simulink model "roll_lqt"  (R2022a)
settings: Solver=ode4  StartTime=0.0  StopTime=26  FixedStep=0.05  RelTol=1e-3
values from neighbouring files (symbols this model uses):
  B = [0 ... (first row only)    [LQR_solver.m]    (also in LQT_solver.m)
  K = ks(1:n, :)    [LQR_solver.m]    (also in LQT_solver.m)
  R_inv = 1    [LQR_solver.m]    (also in LQT_solver.m)
  S = (A' - K * B * R^-1 * B')^-1 * Q    [LQR_solver.m]    (also in LQT_solver.m = K_arr_n(:, 5:end))
settings Model: Creator=Ali  LastModifiedBy=Ali

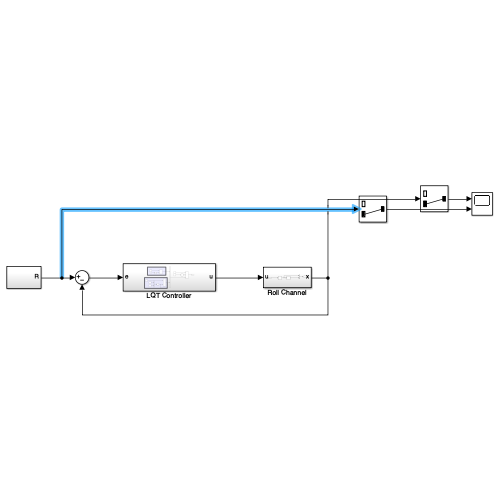
[thumbnail: Simulink's stored preview of the top-level diagram]
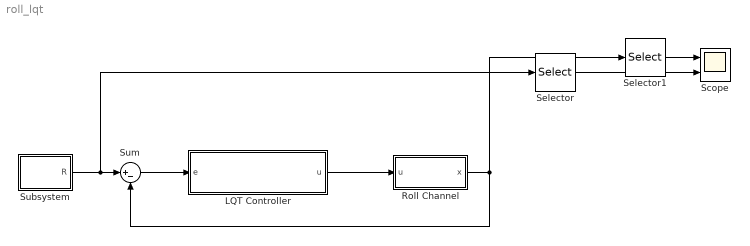
== system roll_lqt ==
  LQT Controller : Subsystem
  Roll Channel : Subsystem
  Scope : Scope  NumInputPorts=2
  Selector : Selector  InputPortWidth=2  IndexOptions=Index vector (dialog)  Indices=[2]  OutputSizes=1
  Selector1 : Selector  InputPortWidth=2  IndexOptions=Index vector (dialog)  Indices=[2]  OutputSizes=1
  Subsystem : Subsystem
  Sum : Sum  Inputs=|+-
  wires:
  LQT Controller/1(u) -> Roll Channel/1(u)
  Subsystem/1(R) -> Selector/1, Sum/1
  Sum/1 -> LQT Controller/1(e)
  Roll Channel/1(x) -> Selector1/1, Sum/2
  Selector1/1 -> Scope/1
  Selector/1 -> Scope/2

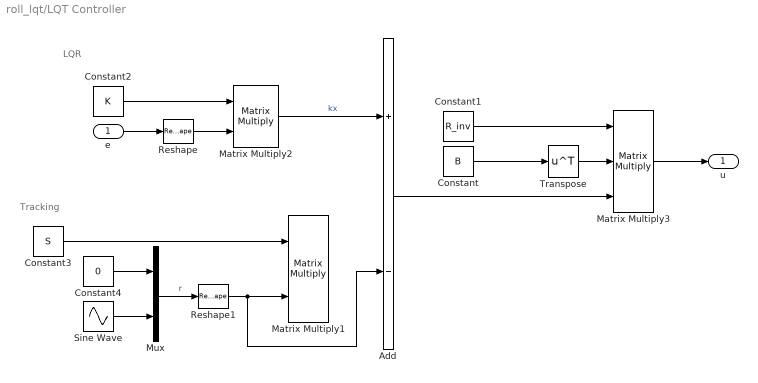
== system roll_lqt/LQT Controller ==
  note: Tracking
  note: LQR
  e : Inport
  Add : Sum  Inputs=+-
  Constant : Constant  Value=B
  Constant1 : Constant  Value=R_inv
  Constant2 : Constant  Value=K
  Constant3 : Constant  Value=S
  Constant4 : Constant  Value=0
  Matrix Multiply1 : Product  Multiplication=Matrix(*)
  Matrix Multiply2 : Product  Multiplication=Matrix(*)
  Matrix Multiply3 : Product  Inputs=3  Multiplication=Matrix(*)
  Mux : Mux  Inputs=2
  Reshape : Reshape  OutputDimensionality=Customize  OutputDimensions=[2,1]
  Reshape1 : Reshape  OutputDimensionality=Customize  OutputDimensions=[2,1]
  Sine Wave : Sin  SampleTime=0
  Transpose : Math  Operator=transpose
  u : Outport
  wires:
  Constant/1 -> Transpose/1
  Constant1/1 -> Matrix Multiply3/1
  Transpose/1 -> Matrix Multiply3/2
  Reshape/1 -> Matrix Multiply2/2
  e/1 -> Reshape/1
  Matrix Multiply3/1 -> u/1
  Constant2/1 -> Matrix Multiply2/1
  Constant4/1 -> Mux/1
  Sine Wave/1 -> Mux/2
  Mux/1 -> Reshape1/1  "r"
  Constant3/1 -> Matrix Multiply1/1
  Reshape1/1 -> Add/2, Matrix Multiply1/2
  Add/1 -> Matrix Multiply3/3
  Matrix Multiply2/1 -> Add/1  "kx"

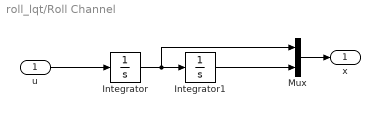
== system roll_lqt/Roll Channel ==
  u : Inport
  Integrator : Integrator
  Integrator1 : Integrator
  Mux : Mux  Inputs=2
  x : Outport
  wires:
  Integrator1/1 -> Mux/2
  u/1 -> Integrator/1
  Integrator/1 -> Mux/1, Integrator1/1
  Mux/1 -> x/1

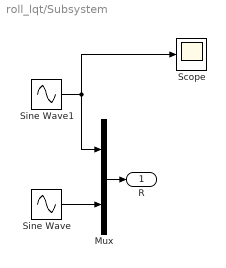
== system roll_lqt/Subsystem ==
  Mux : Mux  Inputs=2
  Scope : Scope
  Sine Wave : Sin  SampleTime=0
  Sine Wave1 : Sin  Phase=pi/2  SampleTime=0
  R : Outport
  wires:
  Mux/1 -> R/1
  Sine Wave/1 -> Mux/2
  Sine Wave1/1 -> Scope/1, Mux/1
